simulink model "TorqueVectoring_6_1"  (R2023a)
settings: Solver=FixedStepAuto  StartTime=0.0  StopTime=8  FixedStep=.001  RelTol=1e-3
model workspace (MAT data in the model file):
  slipTarget = Simulink.Parameter
  slipTarget.Value = 20
  slipTarget.DataType = 'auto'
  slipTarget.Complexity = 'real'
  slipTarget.Dimensions = [1 1]
values from neighbouring files (symbols this model uses):
  Kd_slip = 0    [Main_TorqueVectoring_5_1.m]
  Kd_yaw = 0    [Main_TorqueVectoring_5_1.m]
  Ki_slip = 50    [Main_TorqueVectoring_5_1.m]
  Ki_yaw = 10    [Main_TorqueVectoring_5_1.m]
  Kp_slip = 250    [Main_TorqueVectoring_5_1.m]
  Kp_yaw = 100    [Main_TorqueVectoring_5_1.m]
  slip_windupLower = -inf    [Main_TorqueVectoring_5_1.m]
  slip_windupUpper = inf    [Main_TorqueVectoring_5_1.m]
  slipTarget = .2    (= 0.2)    [Main_TorqueVectoring_5_1.m]
  steering = table2array(yawrateSteering)    [Main_TorqueVectoring_5_1.m]
  yaw_prev_error = 0    [Main_TorqueVectoring_5_1.m]
  yawRate = table2array(yawrateTable)    [Main_TorqueVectoring_5_1.m]
  yawrateVelocity = [0, 5, 10, 15, 20, 25, 30, 35]    [Main_TorqueVectoring_5_1.m]
undefined symbols (not defined in the file or in its folder): sigbuilder_block, VehicleVelocity
libraries: slpidlib x6
(part 1 of 4)
settings Model: Creator=jwong  LastModifiedBy=melis
settings OptimizationCC: ReuseModelBlockBuffer=off
settings DebuggingCC: IgnoredZcDiagnostic=none
settings ModelReferenceCC: EnableRefExpFcnMdlSchedulingChecks=on

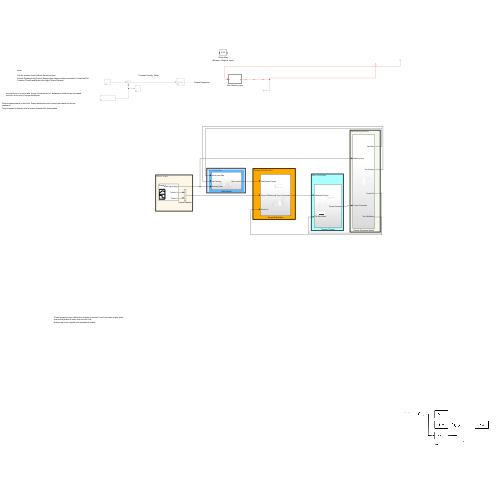
[thumbnail: Simulink's stored preview of the top-level diagram]
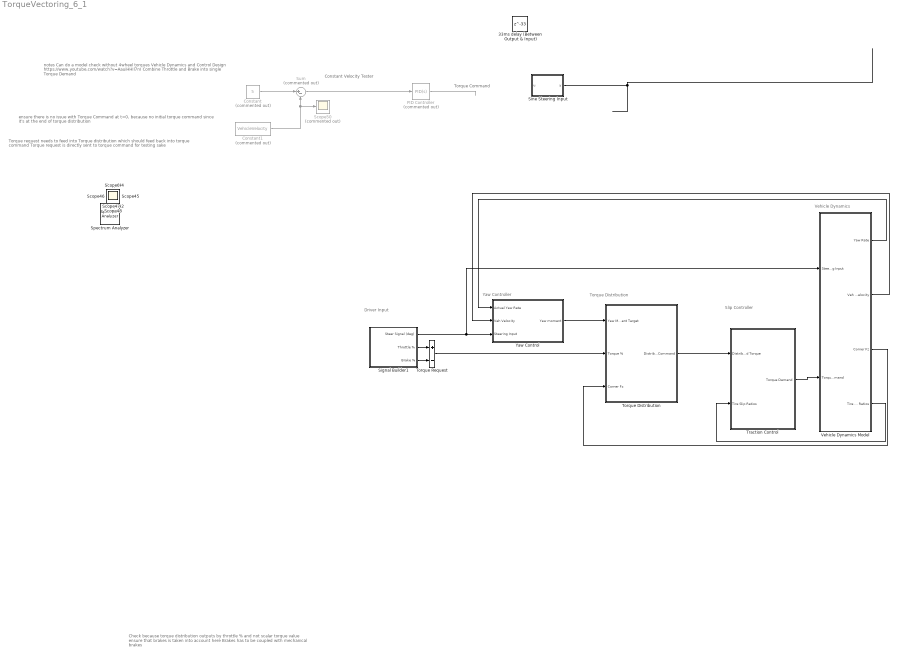
== system TorqueVectoring_6_1 ==
  note: Check because torque distribution outputs by throttle % and not scalar torque value
      | ensure that brakes is taken into account here
      | Brakes has to be coupled with mechanical brakes
  note: Driver Input
  note: Slip Controller
  note: ensure there is no issue with Torque Command at t=0, because no initial torque command since it's at the end of torque distribution
  note: Torque Command
  note: Constant Velocity Tester
  note: Torque request needs to feed into Torque distribution which should feed back into torque command
      | Torque request is directly sent to torque command for testing sake
  note: notes
      |
      | Can do a model check without 4wheel torques
      | Vehicle Dynamics and Control Design https://www.youtube.com/watch?v=AauiHHIl7nI
      | Combine Throttle and Brake into single Torque Demand
  note: Yaw Controller
  note: Torque Distribution
  note: Vehicle Dynamics
  33ms delay (Between Output & Input) : Delay  DelayLength=33
  Constant : Constant  Commented=on  Value=5
  Constant1 : Constant  Commented=on  Value=VehicleVelocity
  PID Controller : slpidlib/PID Controller  Commented=on  Controller=PID  Form=Parallel  TimeDomain=Continuous-time  UseExternalTs=off  SampleTime=-1  IntegratorMethod=Forward Euler  FilterMethod=Forward Euler  ControllerParametersSource=internal  P=1  I=1  UseKiTs=off  D=0  N=100  UseFilter=on  TunerSelectOption=Transfer Function Based (PID Tuner App)  InitialConditionSource=internal  InitialConditionForIntegrator=0  InitialConditionForFilter=0  DifferentiatorICPrevScaledInput=0  ExternalReset=none  TrackingMode=off  Kt=1  LimitOutput=off  SatLimitsSource=internal  UpperSaturationLimit=inf  LowerSaturationLimit=-inf  LinearizeAsGain=on  AntiWindupMode=none  Kb=1  LimitIntegrator=off  UpperIntegratorSaturationLimit=inf  LowerIntegratorSaturationLimit=-inf  POutMin=[]  POutMax=[]  IOutMin=[]  IOutMax=[]  DOutMin=[]  DOutMax=[]  NOutMin=[]  NOutMax=[]  SumOutMin=[]  SumOutMax=[]  SaturationOutMin=[]  SaturationOutMax=[]  PParamMin=[]  PParamMax=[]  IParamMin=[]  IParamMax=[]  DParamMin=[]  DParamMax=[]  NParamMin=[]  NParamMax=[]  KbParamMin=[]  KbParamMax=[]  KtParamMin=[]  KtParamMax=[]  KbOutMin=[]  KbOutMax=[]  KtOutMin=[]  KtOutMax=[]  IntegratorOutMin=[]  IntegratorOutMax=[]  FilterOutMin=[]  FilterOutMax=[]  SumI1OutMin=[]  SumI1OutMax=[]  SumI2OutMin=[]  SumI2OutMax=[]  SumI3OutMin=[]  SumI3OutMax=[]  SumI4OutMin=[]  SumI4OutMax=[]  SumDOutMin=[]  SumDOutMax=[]  DifferentiatorOutMin=[]  DifferentiatorOutMax=[]  FilterDiffOutCoefMin=[]  FilterDiffOutCoefMax=[]  ReciprocalOutMin=[]  ReciprocalOutMax=[]  SumDenOutMin=[]  SumDenOutMax=[]  SumNumOutMin=[]  SumNumOutMax=[]  DivideOutMin=[]  DivideOutMax=[]  UdiffTsProdOutMin=[]  UdiffTsProdOutMax=[]  NTsProdOutMin=[]  NTsProdOutMax=[]  UintegralTsProdOutMin=[]  UintegralTsProdOutMax=[]  UngainTsProdOutMin=[]  UngainTsProdOutMax=[]  ClampingZeroOutDataTypeStr=Inherit: Inherit via back propagation  ClampingZeroOutMin=[]  ClampingZeroOutMax=[]  FilterDenConstantOutDataTypeStr=Inherit: Inherit via back propagation  FilterDenConstantOutMin=[]  FilterDenConstantOutMax=[]  PCopyOutDataTypeStr=Inherit: Inherit via back propagation  PCopyOutMin=[]  PCopyOutMax=[]  NCopyOutDataTypeStr=Inherit: Inherit via back propagation  NCopyOutMin=[]  NCopyOutMax=[]  IntegratorContinuousStateAttributes=''  IntegratorStateMustResolveToSignalObject=off  IntegratorRTWStateStorageClass=Auto  FilterContinuousStateAttributes=''  FilterStateMustResolveToSignalObject=off  FilterRTWStateStorageClass=Auto  ParallelPVariant=InternalParameters  IdealPVariant=Disabled  IVariant=InternalParameters  DVariant=InternalParameters  IntegratorVariant=Continuous  SatVariant=Disabled  AWVariant=Passthrough  PCopyVariant=Disabled  TRVariant=Disabled  FdbkBlocksVariant=Forward  IdealPFdbkVariant=Disabled  SatFdbkVariant=Disabled  DerivativeFilterVariant=ContFilter  NVariant=InternalParameters  NCopyVariant=Disabled  FilterICVariant=InternalICsFilter  IntegratorICVariant=InternalICs  ExternalResetVariant=Disabled  TRSumVariant=Passthrough  SumFdbkVariant=Disabled  SumVariant=Sum_PID  TsampFilterVariant=InternalTs  TsampNgainVariant=Passthrough  TsampIntegralVariant=Disabled_SignalSpec  ExternalSaturationOutDataTypeStr=Inherit: Same as second input
  Scope50 : Scope  Commented=on
  Signal Builder1 : Subsystem  Tag=STV Subsys  LoadFcn=sigbuilder_block('load');  StartFcn=sigbuilder_block('start');  StopFcn=sigbuilder_block('stop');  ClipboardFcn=sigbuilder_block('clipboard');  mask(Sigbuilder block){tuvar=[0:10]}
      mask help: Sigbuilder GUI
      mask init:
      | if ~strcmp(get_param(bdroot(gcbh),'SimulationStatus'),'stopped') tuvar = sigbuilder_block('maskInit'); end
      settings: CopyFcn=sigbuilder_block('copy');  DeleteFcn=sigbuilder_block('delete');  ModelCloseFcn=sigbuilder_block('modelClose');  PreSaveFcn=sigbuilder_block('preSave');  PauseFcn=sigbuilder_block('pause')  ContinueFcn=sigbuilder_block('continue')  NameChangeFcn=sigbuilder_block('namechange');  OpenFcn=sigbuilder_block('open',[120.75 66 1313.25 670.5 ]);  CloseFcn=sigbuilder_block('close');
      mask Display: plot(0, 0, 100, 100,[2, 2, 32, 32, 2], [68, 8, 8, 68, 68],[32, 2], [38, 38], [32, 19, 2],[53, 60, 44], [32, 17, 17, 2],[16, 16, 31, 31]);txt = getActiveGroup(gcbh);text(2, 100, txt,'verticalAlignment', 'top');
  Sine Steering Input : MATLAB Function  TreatAsAtomicUnit=on
  Sum : Sum  Commented=on  Inputs=|+-
  Torque Distribution : Subsystem
  Torque Request : Sum  Inputs=+-
  Traction Control : Subsystem
  Vehicle Dynamics Model : Subsystem
  Yaw Control : Subsystem
  Scope{6,39..48} (11 alike) : Scope
  Spectrum Analyzer : SpectrumAnalyzer  IOType=viewer  WindowPosition=[680 330 560 420]  Method=Welch  SampleRate=10  AveragingMethod=Running
      settings: OpenAtSimulationStart=off
  wires:
  Signal Builder1/1(Steer Signal (deg)) -> Yaw Control/3(Steering Input), Vehicle Dynamics Model/1(Steering Input)
  Signal Builder1/3(Brake %) -> Torque Request/2
  Vehicle Dynamics Model/4(Tire Slip Ratios) -> Traction Control/2(Tire Slip Ratios)
  Vehicle Dynamics Model/1(Yaw Rate) -> Yaw Control/1(Actual Yaw Rate)
  Yaw Control/1(Yaw moment) -> Torque Distribution/1(Yaw Moment Target)
  Traction Control/1(Torque Demand) -> Vehicle Dynamics Model/2(Torque Command)
  Signal Builder1/2(Throttle %) -> Torque Request/1
  Torque Request/1 -> Torque Distribution/2(Torque %)
  Sum/1 -> PID Controller/1
  Constant/1 -> Sum/1
  Vehicle Dynamics Model/2(Veh Velocity) -> Yaw Control/2(Veh Velocity)
  PID Controller/1 -> ?
  Vehicle Dynamics Model/3(Corner Fz) -> Torque Distribution/3(Corner Fz)
  Constant1/1 -> Scope50/1, Sum/2
  ? -> Sine Steering Input/1(u)
  Sine Steering Input/1(y) -> ?
  Torque Distribution/1(Distributed Torque Command) -> Traction Control/1("Distributed Torque ")

== system TorqueVectoring_6_1/Signal Builder1 ==
  Demux : Demux  Tag=STV Demux  Outputs=3
      settings: DisplayOption=none
  FromWs : FromWorkspace  Tag=STV FromWs  VariableName=tuvar
      SigBuilderData=|
      | common.afterFinalStr = 'Extrapolate'
      | common.sampleTime = 0
      | dataSet.timeRange = [0 30]
      | dataSet.name = 'Group 1'
      | sbobj.Name = 'Signal Builder'
      | sbobj.Groups.Name = 'Group 1'
      | sbobj.Groups.Signals(1).Name = 'Steer Signal (deg)'
      | sbobj.Groups.Signals(1).XData = [0 2 2 30]
      | sbobj.Groups.Signals(1).YData = [0 0 20 20]
      | sbobj.Groups.Signals(2).Name = 'Throttle %'
      | sbobj.Groups.Signals(2).XData = [0 2 30]
      | sbobj.Groups.Signals(2).YData = [85 85 85]
      | sbobj.Groups.Signals(3).Name = 'Brake %'
      | sbobj.Groups.Signals(3).XData = [0 5 30]
      | sbobj.Groups.Signals(3).YData = [0 0 0]
      | sbobj.Groups.TimeRange = [0 30]
  Steer Signal (deg) : Outport  Tag=STV Outport
  Throttle % : Outport  Tag=STV Outport  Port=2
  Brake % : Outport  Tag=STV Outport  Port=3
  wires:
  FromWs/1 -> Demux/1
  Demux/1 -> Steer Signal (deg)/1
  Demux/2 -> Throttle %/1
  Demux/3 -> Brake %/1

== system TorqueVectoring_6_1/Torque Distribution ==
  note: Throttle % needs to be checked against look up table and slip control for the maximum torque wheel
  note: output of saturation is the max torque requests for 4 tires, but driver Request is 1 signal
  note: FIX: The input is 4 signal mux of each corner max
  note: saturation can be used to set the limits to allowable torque
  note: Needs to switch based off a corner that has the maximum traction
  note: note
      | make sure this does not limit torque if slip control is not active
  note: note
      | Sum of Moments = (Tfl + Tfr + Trl + Trr)*tw/2/Rw
      | Max allowable torque - every other torque will be a percentage of that torque to = the yaw moment,
      |
      | if traction control = 1
      | torqueOutput = slipcontrolledTorque
      | elseif traction control = 0
      | torqueOutputMax = driverrequested torque% * maxTorqueallowable
      |
      | How to get max torque allowable to one wheel and distribute, by percentage?
      | Send peak torque to highest gripped outside tires, calculate torque that must be offset by other motors
  Yaw Moment Target : Inport
  Torque % : Inport  Port=2
  Corner Fz : Inport  Port=3
  Demux : Demux
  Front-Rear Bias : MATLAB Function  TreatAsAtomicUnit=on
  MATLAB Function : MATLAB Function  Commented=on  TreatAsAtomicUnit=on
  Mux : Mux
  Percentage : Gain  Gain=.01
  To Workspace1 : ToWorkspace  VariableName=distributedtorqueFL  SampleTime=-1
  To Workspace2 : ToWorkspace  VariableName=distributedtorqueFR  SampleTime=-1
  To Workspace3 : ToWorkspace  VariableName=distributedtorqueRL  SampleTime=-1
  To Workspace4 : ToWorkspace  VariableName=distributedtorqueRR  SampleTime=-1
  To Workspace9 : ToWorkspace  VariableName=TorquePer  SaveFormat=Timeseries  SampleTime=-1
  Torque Distribution : MATLAB Function  TreatAsAtomicUnit=on
  Distributed Torque Command : Outport
  wires:
  Yaw Moment Target/1 -> Torque Distribution/1(Mz)
  Corner Fz/1 -> Demux/1
  Demux/1 -> Front-Rear Bias/1(zFL)
  Demux/2 -> Front-Rear Bias/2(zFR)
  Demux/3 -> Front-Rear Bias/3(zRL)
  Demux/4 -> Front-Rear Bias/4(zRR)
  Front-Rear Bias/1(lambda) -> Torque Distribution/3(lambda)
  Torque %/1 -> Percentage/1
  Torque Distribution/2(FRtorque) -> To Workspace2/1, Mux/2
  Torque Distribution/3(RLtorque) -> To Workspace3/1, Mux/3
  Percentage/1 -> To Workspace9/1, Torque Distribution/2(torquePer)
  Mux/1 -> Distributed Torque Command/1
  Torque Distribution/1(FLtorque) -> To Workspace1/1, Mux/1
  Torque Distribution/4(RRtorque) -> To Workspace4/1, Mux/4

== system TorqueVectoring_6_1/Traction Control ==
  note: Outputs are converted to torque instead of tractive force because VCU will command torque setpoints to the inverters
  note: note
      | can bias front to have less torque output @ acceleration to ensure slip ratio and vice versa
  note: Torques must be split here because each tire has their own feedback
  note: note
      | if |slip ratio| > slip ratio target
      | Max allowable torque would be fed from lookup tables
  note: note
      | Does 4 PID Controllers make sense here?
      | Yes - slip control at each individual wheel depending on their indivudal slip
      | Does the PID output a torque command here?
      | Need slip ratio to work under braking - slip ratio target needs to be upper and lower bound
      | if torque command is negative, slip ratio target =-2
      | slip ratio is negative, cannot be > -2
  note: Slip target is a parameter variable of Model workspace
      | *see Model Explorer
  note: **Look up tables can be an an issue when slip ratio is 0 and therefore produces no load
  note: **Ensure Lookup tables can handle negative direction
  "Distributed Torque " : Inport
  Tire Slip Ratios : Inport  Port=2
  Add : Sum
  Demux : Demux
  FL : Subsystem
  FR : Subsystem
  Gain1 : Gain  Gain=1/1.2
  Mux : Mux
  RL : Subsystem
  RR : Subsystem
  Slip Target Constant : Constant  Value=slipTarget
  To Workspace4 : ToWorkspace  VariableName=torqueDemand  SampleTime=-1
  Torque Demand : Outport
  wires:
  Demux/1 -> FL/1(slip Ratio)
  Demux/2 -> FR/1(slip Ratio)
  Demux/3 -> RL/1(slip Ratio)
  Demux/4 -> RR/1(slip Ratio)
  Mux/1 -> Add/2, To Workspace4/1
  FL/1(Allowable Torque) -> Mux/1  "FL PID torque adjust"
  FR/1(Allowable Torque) -> Mux/2  "FR PID torque  adjust"
  RL/1(Allowable Torque) -> Mux/3  "RL PID torque adjust"
  RR/1(Allowable Torque) -> Mux/4  "RR PID torque  adjust"
  Slip Target Constant/1 -> RR/2(slipTarget), RL/2(slipTarget), FR/2(slipTarget), FL/2(slipTarget)
  Add/1 -> Torque Demand/1
  "Distributed Torque "/1 -> Add/1
  Tire Slip Ratios/1 -> Gain1/1
  Gain1/1 -> Demux/1

== system TorqueVectoring_6_1/Vehicle Dynamics Model ==
  note: Tire slipAngles not used to calculate Fy, not accurate enough sensors for real use
  Steering Input : Inport
  Torque Command : Inport  Port=2
  " Slip Angles" : Mux  Commented=on
  " Slip Ratios" : Mux
  14 DOF MODEL : Subsystem  mask{Ms=180.9, a=0.8169783, b=0.707009, wf=1.34, wr=1.34, h=0.23, mt=241.7, Lf=.64, Lr=.88392, Ip=64.46, Ir=15.34, Jz=70.38, mufl=7.4, mufr=7.4, murl=7.8, murr=7.8, Rw=.4064, Iw=3.033213, Ksfl=19.3, Ksfr=19.3, Ksrl=24.8, Ksrr=24.8, Csfl=1437.611, Csfr=1437.611, Csrl=1644.42, Csrr=1644.42, Ktfl=113832.44275, Ktfr=113832.44275, Ktrl=113832.44275, Ktrr=113832.44275, g=9.8}
      mask prompts: Ms "Vehicle sprung mass (kg)"; a "Distance of sprung mass C.G. from front axle (m)"; b "Distance of sprung mass C.G. from rear axle (m)"; wf "Front track width (m)"; wr "Rear track width (m)"; h "Height of sprung mass C.G. from rground (m)"; mt "Vehicle total mass (kg)"; Lf "Distance of vehicle C.G. from front axle (m)"; Lr "Distance of vehicle C.G. from rear axle (m)"; Ip "Pitch moment of inertia (kgm^2)"; Ir "Roll moment of inertia (kgm^2)"; Jz "Yaw moment of inertia (kgm^2)"; mufl "Front left unsprung mass (kg)"; mufr "Front right unsprung mass (kg)"; murl "Rear left unsprung mass (kg)"; murr "Rear right unsprung mass (kg)"; Rw "Wheel radius (m)"; Iw "Wheel moment of inertia (kgm^2)"; Ksfl "Front left suspension stiffness (N/m)"; Ksfr "Front right suspension stiffness (N/m)"; Ksrl "Rear left suspension stiffness (N/m)"; Ksrr "Rear right suspension stiffness (N/m)"; Csfl "Front left suspension damping coefficient (Nsec/m)"; Csfr "Front right suspension damping coefficient (Nsec/m)"; Csrl "Rear left suspension damping coefficient (Nsec/m)"; Csrr "Rear right suspension damping coefficient (Nsec/m)"; Ktfl "Front left tire stiffness (N/m)"; Ktfr "Front right tire stiffness (N/m)"; Ktrl "Rear left tire stiffness (N/m)"; Ktrr "Rear right tire stiffness (N/m)"; g "Gravitational acceleration (ms^-2)"
      mask Display: %image(imread('E:\Google Drive\FSAE Electric\In Hub Motors Torque Vectoring Masters Project\Simulink\IMG_8647.JPG'))
  Constant : Constant  Value=.001
  Demux : Demux
  Gain : Gain
  Gain1 : Gain  Gain=1/1000
  Radians to deg : Gain  Gain=57.2958
  Scope : Scope
  Signal Builder : Subsystem  Tag=STV Subsys  LoadFcn=sigbuilder_block('load');  StartFcn=sigbuilder_block('start');  StopFcn=sigbuilder_block('stop');  ClipboardFcn=sigbuilder_block('clipboard');  mask(Sigbuilder block){tuvar=[0:10]}
      mask help: Simulink:masks:SigbuilderBlock_MD
      mask init:
      | if ~strcmp(get_param(bdroot(gcbh),'SimulationStatus'),'stopped') tuvar = sigbuilder_block('maskInit'); end
      settings: CopyFcn=sigbuilder_block('copy');  DeleteFcn=sigbuilder_block('delete');  ModelCloseFcn=sigbuilder_block('modelClose');  PreSaveFcn=sigbuilder_block('preSave');  PauseFcn=sigbuilder_block('pause');  ContinueFcn=sigbuilder_block('continue');  NameChangeFcn=sigbuilder_block('namechange');  OpenFcn=sigbuilder_block('open',[437.6 199.2 550.4 400 ]);  CloseFcn=sigbuilder_block('close');
      mask Display: plot(0, 0, 100, 100,[2, 2, 32, 32, 2], [68, 8, 8, 68, 68],[32, 2], [38, 38], [32, 19, 2],[53, 60, 44], [32, 17, 17, 2],[16, 16, 31, 31]);txt = getActiveGroup(gcbh);text(2, 100, txt,'verticalAlignment', 'top');
  To Workspace : ToWorkspace  VariableName=LatAcc  SampleTime=-1
  To Workspace1 : ToWorkspace  VariableName=YawRate  SampleTime=-1
  To Workspace5 : ToWorkspace  VariableName=T_FL  SampleTime=-1
  To Workspace6 : ToWorkspace  VariableName=T_FR  SampleTime=-1
  To Workspace7 : ToWorkspace  VariableName=T_RL  SampleTime=-1
  To Workspace8 : ToWorkspace  VariableName=T_RR  SampleTime=-1
  X Position : ToWorkspace  VariableName=X  SampleTime=-1
  Y Position : ToWorkspace  VariableName=Y  SampleTime=-1
  fl Slip : ToWorkspace  VariableName=FLsr  SampleTime=-1
  fl slip angle : Scope
  fr Slip : ToWorkspace  VariableName=FRsr  SampleTime=-1
  fr slip angle : Scope
  lateral acceleration : Scope
  rl Slip : ToWorkspace  VariableName=RLsr  SampleTime=-1
  rl slip angle : Scope
  roll angle : Scope
  rr Slip : ToWorkspace  VariableName=RRsr  SampleTime=-1
  rr slip angle : Scope
  steering : Scope
  yaw rate : Scope
  Yaw Rate : Outport
  Veh Velocity : Outport  Port=2
  Corner Fz : Outport  Port=3
  Tire Slip Ratios : Outport  Port=4
  wires:
  14 DOF MODEL/3(roll angle) -> roll angle/1
  14 DOF MODEL/1(ay) -> To Workspace/1, lateral acceleration/1
  Gain/1 -> 14 DOF MODEL/1(steer)
  14 DOF MODEL/9(Y) -> Y Position/1  "Ypos"
  14 DOF MODEL/8(X) -> X Position/1  "Xpos"
  Steering Input/1 -> steering/1, Gain/1
  14 DOF MODEL/2(yaw rate) -> Radians to deg/1
  14 DOF MODEL/4(fl slip angle) -> " Slip Angles"/1, fl slip angle/1
  14 DOF MODEL/5(fr slip angle) -> " Slip Angles"/2, fr slip angle/1
  14 DOF MODEL/6(rl slip angle) -> " Slip Angles"/3, rl slip angle/1
  14 DOF MODEL/7(rr slip angle) -> " Slip Angles"/4, rr slip angle/1
  14 DOF MODEL/11(fr Slip Ratio) -> fr Slip/1, " Slip Ratios"/2  "fr SlipRatio"
  14 DOF MODEL/12(rl Slip Ratio) -> " Slip Ratios"/3, rl Slip/1  "rl SlipRatio"
  " Slip Ratios"/1 -> Gain1/1
  14 DOF MODEL/10(fl Slip Ratio) -> fl Slip/1, " Slip Ratios"/1  "fl SlipRatio"
  14 DOF MODEL/13(rr Slip Ratio) -> rr Slip/1, " Slip Ratios"/4  "rr SlipRatio"
  " Slip Angles"/1 -> ?
  Torque Command/1 -> Demux/1, Scope/1
  Constant/1 -> 14 DOF MODEL/2(Vx (Initial))
  Radians to deg/1 -> Yaw Rate/1, yaw rate/1, To Workspace1/1  "deg"
  14 DOF MODEL/14(Veh Velocity) -> Veh Velocity/1
  14 DOF MODEL/15(Corner Fz) -> Corner Fz/1
  Demux/3 -> To Workspace7/1, 14 DOF MODEL/5(TaRL)
  Demux/2 -> To Workspace6/1, 14 DOF MODEL/4(TaFR)
  Demux/4 -> To Workspace8/1, 14 DOF MODEL/6(TaRR)
  Demux/1 -> To Workspace5/1, 14 DOF MODEL/3(TaFL)
  Gain1/1 -> Tire Slip Ratios/1

== system TorqueVectoring_6_1/Yaw Control ==
  Actual Yaw Rate : Inport
  Veh Velocity : Inport  Port=2
  Steering Input : Inport  Port=3
  Abs : Abs  SaturateOnIntegerOverflow=off
  Add : Sum
  Constant : Constant  Value=.001
  Constant1 : Constant  Value=10
  Constant2 : Constant  Value=-1
  Gain : Gain  Gain=1.6180217600198381947242800905118
  MATLAB Function : MATLAB Function  TreatAsAtomicUnit=on
  PID Controller : slpidlib/PID Controller  Commented=on  Controller=PID  Form=Parallel  TimeDomain=Discrete-time  UseExternalTs=off  SampleTime=-1  IntegratorMethod=Backward Euler  FilterMethod=Backward Euler  ControllerParametersSource=internal  P=Kp_yaw  I=Ki_yaw  UseKiTs=off  D=Kd_yaw  N=100  UseFilter=on  TunerSelectOption=Frequency Response Based  InitialConditionSource=internal  InitialConditionForIntegrator=0  InitialConditionForFilter=0  DifferentiatorICPrevScaledInput=0  ExternalReset=none  TrackingMode=off  Kt=1  LimitOutput=on  SatLimitsSource=internal  UpperSaturationLimit=inf  LowerSaturationLimit=-inf  LinearizeAsGain=on  AntiWindupMode=clamping  Kb=1  LimitIntegrator=off  UpperIntegratorSaturationLimit=inf  LowerIntegratorSaturationLimit=-inf  POutMin=[]  POutMax=[]  IOutMin=[]  IOutMax=[]  DOutMin=[]  DOutMax=[]  NOutMin=[]  NOutMax=[]  SumOutMin=[]  SumOutMax=[]  SaturationOutMin=[]  SaturationOutMax=[]  PParamMin=[]  PParamMax=[]  IParamMin=[]  IParamMax=[]  DParamMin=[]  DParamMax=[]  NParamMin=[]  NParamMax=[]  KbParamMin=[]  KbParamMax=[]  KtParamMin=[]  KtParamMax=[]  KbOutMin=[]  KbOutMax=[]  KtOutMin=[]  KtOutMax=[]  IntegratorOutMin=[]  IntegratorOutMax=[]  FilterOutMin=[]  FilterOutMax=[]  SumI1OutMin=[]  SumI1OutMax=[]  SumI2OutMin=[]  SumI2OutMax=[]  SumI3OutMin=[]  SumI3OutMax=[]  SumI4OutMin=[]  SumI4OutMax=[]  SumDOutMin=[]  SumDOutMax=[]  DifferentiatorOutMin=[]  DifferentiatorOutMax=[]  FilterDiffOutCoefMin=[]  FilterDiffOutCoefMax=[]  ReciprocalOutMin=[]  ReciprocalOutMax=[]  SumDenOutMin=[]  SumDenOutMax=[]  SumNumOutMin=[]  SumNumOutMax=[]  DivideOutMin=[]  DivideOutMax=[]  UdiffTsProdOutMin=[]  UdiffTsProdOutMax=[]  NTsProdOutMin=[]  NTsProdOutMax=[]  UintegralTsProdOutMin=[]  UintegralTsProdOutMax=[]  UngainTsProdOutMin=[]  UngainTsProdOutMax=[]  ClampingZeroOutDataTypeStr=Inherit: Inherit via back propagation  ClampingZeroOutMin=[]  ClampingZeroOutMax=[]  FilterDenConstantOutDataTypeStr=Inherit: Inherit via back propagation  FilterDenConstantOutMin=[]  FilterDenConstantOutMax=[]  PCopyOutDataTypeStr=Inherit: Inherit via back propagation  PCopyOutMin=[]  PCopyOutMax=[]  NCopyOutDataTypeStr=Inherit: Inherit via back propagation  NCopyOutMin=[]  NCopyOutMax=[]  IntegratorContinuousStateAttributes=''  IntegratorStateMustResolveToSignalObject=off  IntegratorRTWStateStorageClass=Auto  FilterContinuousStateAttributes=''  FilterStateMustResolveToSignalObject=off  FilterRTWStateStorageClass=Auto  ParallelPVariant=InternalParameters  IdealPVariant=Disabled  IVariant=InternalParameters  DVariant=InternalParameters  IntegratorVariant=Discrete  SatVariant=Enabled  AWVariant=DiscClampingParallel  PCopyVariant=Disabled  TRVariant=Disabled  FdbkBlocksVariant=Feedback  IdealPFdbkVariant=Passthrough  SatFdbkVariant=Passthrough  DerivativeFilterVariant=BackwardEulerFilter  NVariant=InternalParameters  NCopyVariant=InternalParameters  FilterICVariant=InternalICsFilter  IntegratorICVariant=InternalICs  ExternalResetVariant=Disabled  TRSumVariant=Passthrough  SumFdbkVariant=Enabled  SumVariant=Sum_PID  TsampFilterVariant=InternalTs  TsampNgainVariant=Passthrough  TsampIntegralVariant=Disabled_SignalSpec  ExternalSaturationOutDataTypeStr=Inherit: Same as second input
  Product2 : Product
  Steering vs Velocity Yaw Rate Lookup Table : Lookup_n-D  BreakpointsForDimension1=steering  BreakpointsForDimension2=yawrateVelocity  Table=yawRate  InternalRulePriority=Speed  RndMeth=Simplest
      settings: InputPortMap=u0,u1
  Sum : Sum  Inputs=|+-
  Switch : Switch  Criteria=u2 > Threshold  ZeroCross=off  SaturateOnIntegerOverflow=off  InputSameDT=off
  To Workspace : ToWorkspace  VariableName=steeringAngle  SaveFormat=Timeseries  SampleTime=-1
  To Workspace1 : ToWorkspace  VariableName=YawRateSetpoint  SaveFormat=Timeseries  SampleTime=-1
  To Workspace2 : ToWorkspace  VariableName=YawMomentTarget  SaveFormat=Timeseries  SampleTime=-1
  To Workspace3 : ToWorkspace  VariableName=YawRateError  SaveFormat=Timeseries  SampleTime=-1
  Yaw moment : Outport
  wires:
  Steering Input/1 -> To Workspace/1, Switch/2, Product2/1, Abs/1
  Sum/1 -> To Workspace3/1, MATLAB Function/1(yaw_error)  "Yaw Rate Error"
  Veh Velocity/1 -> Add/1
  Steering vs Velocity Yaw Rate Lookup Table/1 -> Gain/1  "Yaw Rate  Setpoint"
  Add/1 -> Steering vs Velocity Yaw Rate Lookup Table/2
  Constant/1 -> Add/2
  Abs/1 -> Steering vs Velocity Yaw Rate Lookup Table/1
  Constant2/1 -> Product2/2
  Product2/1 -> Switch/3
  Switch/1 -> Yaw moment/1
  Actual Yaw Rate/1 -> Sum/2
  Gain/1 -> To Workspace1/1, Sum/1
  MATLAB Function/1(yaw_target) -> To Workspace2/1, Switch/1

== system TorqueVectoring_6_1/Traction Control/FL ==
  slip Ratio : Inport
  slipTarget : Inport  Port=2
  Constant : Constant  Value=0
  MATLAB Function : MATLAB Function  TreatAsAtomicUnit=on
  PID Controller5 : slpidlib/PID Controller  Controller=PID  Form=Parallel  TimeDomain=Continuous-time  UseExternalTs=off  SampleTime=-1  IntegratorMethod=Forward Euler  FilterMethod=Forward Euler  ControllerParametersSource=internal  P=Kp_slip  I=Ki_slip  UseKiTs=off  D=Kd_slip  N=100  UseFilter=on  TunerSelectOption=Transfer Function Based (PID Tuner App)  ZeroCross=off  InitialConditionSource=internal  InitialConditionForIntegrator=0  InitialConditionForFilter=0  DifferentiatorICPrevScaledInput=0  ExternalReset=none  TrackingMode=off  Kt=1  LimitOutput=off  SatLimitsSource=internal  UpperSaturationLimit=slip_windupUpper  LowerSaturationLimit=slip_windupLower  LinearizeAsGain=on  AntiWindupMode=clamping  Kb=1  LimitIntegrator=off  UpperIntegratorSaturationLimit=inf  LowerIntegratorSaturationLimit=-inf  POutMin=[]  POutMax=[]  IOutMin=[]  IOutMax=[]  DOutMin=[]  DOutMax=[]  NOutMin=[]  NOutMax=[]  SumOutMin=[]  SumOutMax=[]  SaturationOutMin=[]  SaturationOutMax=[]  PParamMin=[]  PParamMax=[]  IParamMin=[]  IParamMax=[]  DParamMin=[]  DParamMax=[]  NParamMin=[]  NParamMax=[]  KbParamMin=[]  KbParamMax=[]  KtParamMin=[]  KtParamMax=[]  KbOutMin=[]  KbOutMax=[]  KtOutMin=[]  KtOutMax=[]  IntegratorOutMin=[]  IntegratorOutMax=[]  FilterOutMin=[]  FilterOutMax=[]  SumI1OutMin=[]  SumI1OutMax=[]  SumI2OutMin=[]  SumI2OutMax=[]  SumI3OutMin=[]  SumI3OutMax=[]  SumI4OutMin=[]  SumI4OutMax=[]  SumDOutMin=[]  SumDOutMax=[]  DifferentiatorOutMin=[]  DifferentiatorOutMax=[]  FilterDiffOutCoefMin=[]  FilterDiffOutCoefMax=[]  ReciprocalOutMin=[]  ReciprocalOutMax=[]  SumDenOutMin=[]  SumDenOutMax=[]  SumNumOutMin=[]  SumNumOutMax=[]  DivideOutMin=[]  DivideOutMax=[]  UdiffTsProdOutMin=[]  UdiffTsProdOutMax=[]  NTsProdOutMin=[]  NTsProdOutMax=[]  UintegralTsProdOutMin=[]  UintegralTsProdOutMax=[]  UngainTsProdOutMin=[]  UngainTsProdOutMax=[]  ClampingZeroOutDataTypeStr=Inherit: Inherit via back propagation  ClampingZeroOutMin=[]  ClampingZeroOutMax=[]  FilterDenConstantOutDataTypeStr=Inherit: Inherit via back propagation  FilterDenConstantOutMin=[]  FilterDenConstantOutMax=[]  PCopyOutDataTypeStr=Inherit: Inherit via back propagation  PCopyOutMin=[]  PCopyOutMax=[]  NCopyOutDataTypeStr=Inherit: Inherit via back propagation  NCopyOutMin=[]  NCopyOutMax=[]  IntegratorContinuousStateAttributes=''  IntegratorStateMustResolveToSignalObject=off  IntegratorRTWStateStorageClass=Auto  FilterContinuousStateAttributes=''  FilterStateMustResolveToSignalObject=off  FilterRTWStateStorageClass=Auto  ParallelPVariant=InternalParameters  IdealPVariant=Disabled  IVariant=InternalParameters  DVariant=InternalParameters  IntegratorVariant=Continuous  SatVariant=Disabled  AWVariant=Passthrough  PCopyVariant=Disabled  TRVariant=Disabled  FdbkBlocksVariant=Forward  IdealPFdbkVariant=Disabled  SatFdbkVariant=Disabled  DerivativeFilterVariant=ContFilter  NVariant=InternalParameters  NCopyVariant=Disabled  FilterICVariant=InternalICsFilter  IntegratorICVariant=InternalICs  ExternalResetVariant=Disabled  TRSumVariant=Passthrough  SumFdbkVariant=Disabled  SumVariant=Sum_PID  TsampFilterVariant=InternalTs  TsampNgainVariant=Passthrough  TsampIntegralVariant=Disabled_SignalSpec  ExternalSaturationOutDataTypeStr=Inherit: Same as second input
  Scope : Scope
  Scope1 : Scope
  Sum5 : Sum  Inputs=|+-
  Switch : Switch  Criteria=u2 > Threshold  ZeroCross=off  SaturateOnIntegerOverflow=off  InputSameDT=off
  To Workspace1 : ToWorkspace  VariableName=FLslipError  SaveFormat=Timeseries  SampleTime=-1
  fl Slip : ToWorkspace  VariableName=FLsr1  SampleTime=-1
  Allowable Torque : Outport
  wires:
  MATLAB Function/2(setpoint) -> Sum5/1
  Sum5/1 -> To Workspace1/1, PID Controller5/1  "slip error"
  Switch/1 -> Allowable Torque/1
  slip Ratio/1 -> fl Slip/1, MATLAB Function/1(actualSlip), Sum5/2
  slipTarget/1 -> MATLAB Function/2(SlipTarget)
  MATLAB Function/1(enable) -> Switch/2, Scope/1
  PID Controller5/1 -> Scope1/1, Switch/1
  Constant/1 -> Switch/3

== system TorqueVectoring_6_1/Traction Control/FR ==
  slip Ratio : Inport
  slipTarget : Inport  Port=2
  Constant : Constant  Value=0
  MATLAB Function : MATLAB Function  TreatAsAtomicUnit=on
  PID Controller5 : slpidlib/PID Controller  Controller=PID  Form=Parallel  TimeDomain=Continuous-time  UseExternalTs=off  SampleTime=-1  IntegratorMethod=Forward Euler  FilterMethod=Forward Euler  ControllerParametersSource=internal  P=Kp_slip  I=Ki_slip  UseKiTs=off  D=Kd_slip  N=100  UseFilter=on  TunerSelectOption=Transfer Function Based (PID Tuner App)  ZeroCross=off  InitialConditionSource=internal  InitialConditionForIntegrator=0  InitialConditionForFilter=0  DifferentiatorICPrevScaledInput=0  ExternalReset=none  TrackingMode=off  Kt=1  LimitOutput=off  SatLimitsSource=internal  UpperSaturationLimit=slip_windupUpper  LowerSaturationLimit=slip_windupLower  LinearizeAsGain=on  AntiWindupMode=clamping  Kb=1  LimitIntegrator=off  UpperIntegratorSaturationLimit=inf  LowerIntegratorSaturationLimit=-inf  POutMin=[]  POutMax=[]  IOutMin=[]  IOutMax=[]  DOutMin=[]  DOutMax=[]  NOutMin=[]  NOutMax=[]  SumOutMin=[]  SumOutMax=[]  SaturationOutMin=[]  SaturationOutMax=[]  PParamMin=[]  PParamMax=[]  IParamMin=[]  IParamMax=[]  DParamMin=[]  DParamMax=[]  NParamMin=[]  NParamMax=[]  KbParamMin=[]  KbParamMax=[]  KtParamMin=[]  KtParamMax=[]  KbOutMin=[]  KbOutMax=[]  KtOutMin=[]  KtOutMax=[]  IntegratorOutMin=[]  IntegratorOutMax=[]  FilterOutMin=[]  FilterOutMax=[]  SumI1OutMin=[]  SumI1OutMax=[]  SumI2OutMin=[]  SumI2OutMax=[]  SumI3OutMin=[]  SumI3OutMax=[]  SumI4OutMin=[]  SumI4OutMax=[]  SumDOutMin=[]  SumDOutMax=[]  DifferentiatorOutMin=[]  DifferentiatorOutMax=[]  FilterDiffOutCoefMin=[]  FilterDiffOutCoefMax=[]  ReciprocalOutMin=[]  ReciprocalOutMax=[]  SumDenOutMin=[]  SumDenOutMax=[]  SumNumOutMin=[]  SumNumOutMax=[]  DivideOutMin=[]  DivideOutMax=[]  UdiffTsProdOutMin=[]  UdiffTsProdOutMax=[]  NTsProdOutMin=[]  NTsProdOutMax=[]  UintegralTsProdOutMin=[]  UintegralTsProdOutMax=[]  UngainTsProdOutMin=[]  UngainTsProdOutMax=[]  ClampingZeroOutDataTypeStr=Inherit: Inherit via back propagation  ClampingZeroOutMin=[]  ClampingZeroOutMax=[]  FilterDenConstantOutDataTypeStr=Inherit: Inherit via back propagation  FilterDenConstantOutMin=[]  FilterDenConstantOutMax=[]  PCopyOutDataTypeStr=Inherit: Inherit via back propagation  PCopyOutMin=[]  PCopyOutMax=[]  NCopyOutDataTypeStr=Inherit: Inherit via back propagation  NCopyOutMin=[]  NCopyOutMax=[]  IntegratorContinuousStateAttributes=''  IntegratorStateMustResolveToSignalObject=off  IntegratorRTWStateStorageClass=Auto  FilterContinuousStateAttributes=''  FilterStateMustResolveToSignalObject=off  FilterRTWStateStorageClass=Auto  ParallelPVariant=InternalParameters  IdealPVariant=Disabled  IVariant=InternalParameters  DVariant=InternalParameters  IntegratorVariant=Continuous  SatVariant=Disabled  AWVariant=Passthrough  PCopyVariant=Disabled  TRVariant=Disabled  FdbkBlocksVariant=Forward  IdealPFdbkVariant=Disabled  SatFdbkVariant=Disabled  DerivativeFilterVariant=ContFilter  NVariant=InternalParameters  NCopyVariant=Disabled  FilterICVariant=InternalICsFilter  IntegratorICVariant=InternalICs  ExternalResetVariant=Disabled  TRSumVariant=Passthrough  SumFdbkVariant=Disabled  SumVariant=Sum_PID  TsampFilterVariant=InternalTs  TsampNgainVariant=Passthrough  TsampIntegralVariant=Disabled_SignalSpec  ExternalSaturationOutDataTypeStr=Inherit: Same as second input
  Scope : Scope
  Scope1 : Scope
  Sum5 : Sum  Inputs=|+-
  Switch : Switch  Criteria=u2 > Threshold  ZeroCross=off  SaturateOnIntegerOverflow=off  InputSameDT=off
  To Workspace1 : ToWorkspace  VariableName=FRslipError  SaveFormat=Timeseries  SampleTime=-1
  fl Slip : ToWorkspace  VariableName=FRsr1  SampleTime=-1
  Allowable Torque : Outport
  wires:
  Constant/1 -> Switch/3
  slipTarget/1 -> MATLAB Function/2(SlipTarget)
  MATLAB Function/1(enable) -> Switch/2, Scope/1
  slip Ratio/1 -> fl Slip/1, MATLAB Function/1(actualSlip), Sum5/2
  Switch/1 -> Allowable Torque/1
  MATLAB Function/2(setpoint) -> Sum5/1
  Sum5/1 -> To Workspace1/1, PID Controller5/1  "slip error"
  PID Controller5/1 -> Scope1/1, Switch/1

== system TorqueVectoring_6_1/Traction Control/RL ==
  slip Ratio : Inport
  slipTarget : Inport  Port=2
  Constant : Constant  Value=0
  MATLAB Function : MATLAB Function  TreatAsAtomicUnit=on
  PID Controller5 : slpidlib/PID Controller  Controller=PID  Form=Parallel  TimeDomain=Continuous-time  UseExternalTs=off  SampleTime=-1  IntegratorMethod=Forward Euler  FilterMethod=Forward Euler  ControllerParametersSource=internal  P=Kp_slip  I=Ki_slip  UseKiTs=off  D=Kd_slip  N=100  UseFilter=on  TunerSelectOption=Transfer Function Based (PID Tuner App)  ZeroCross=off  InitialConditionSource=internal  InitialConditionForIntegrator=0  InitialConditionForFilter=0  DifferentiatorICPrevScaledInput=0  ExternalReset=none  TrackingMode=off  Kt=1  LimitOutput=off  SatLimitsSource=internal  UpperSaturationLimit=slip_windupUpper  LowerSaturationLimit=slip_windupLower  LinearizeAsGain=on  AntiWindupMode=clamping  Kb=1  LimitIntegrator=off  UpperIntegratorSaturationLimit=inf  LowerIntegratorSaturationLimit=-inf  POutMin=[]  POutMax=[]  IOutMin=[]  IOutMax=[]  DOutMin=[]  DOutMax=[]  NOutMin=[]  NOutMax=[]  SumOutMin=[]  SumOutMax=[]  SaturationOutMin=[]  SaturationOutMax=[]  PParamMin=[]  PParamMax=[]  IParamMin=[]  IParamMax=[]  DParamMin=[]  DParamMax=[]  NParamMin=[]  NParamMax=[]  KbParamMin=[]  KbParamMax=[]  KtParamMin=[]  KtParamMax=[]  KbOutMin=[]  KbOutMax=[]  KtOutMin=[]  KtOutMax=[]  IntegratorOutMin=[]  IntegratorOutMax=[]  FilterOutMin=[]  FilterOutMax=[]  SumI1OutMin=[]  SumI1OutMax=[]  SumI2OutMin=[]  SumI2OutMax=[]  SumI3OutMin=[]  SumI3OutMax=[]  SumI4OutMin=[]  SumI4OutMax=[]  SumDOutMin=[]  SumDOutMax=[]  DifferentiatorOutMin=[]  DifferentiatorOutMax=[]  FilterDiffOutCoefMin=[]  FilterDiffOutCoefMax=[]  ReciprocalOutMin=[]  ReciprocalOutMax=[]  SumDenOutMin=[]  SumDenOutMax=[]  SumNumOutMin=[]  SumNumOutMax=[]  DivideOutMin=[]  DivideOutMax=[]  UdiffTsProdOutMin=[]  UdiffTsProdOutMax=[]  NTsProdOutMin=[]  NTsProdOutMax=[]  UintegralTsProdOutMin=[]  UintegralTsProdOutMax=[]  UngainTsProdOutMin=[]  UngainTsProdOutMax=[]  ClampingZeroOutDataTypeStr=Inherit: Inherit via back propagation  ClampingZeroOutMin=[]  ClampingZeroOutMax=[]  FilterDenConstantOutDataTypeStr=Inherit: Inherit via back propagation  FilterDenConstantOutMin=[]  FilterDenConstantOutMax=[]  PCopyOutDataTypeStr=Inherit: Inherit via back propagation  PCopyOutMin=[]  PCopyOutMax=[]  NCopyOutDataTypeStr=Inherit: Inherit via back propagation  NCopyOutMin=[]  NCopyOutMax=[]  IntegratorContinuousStateAttributes=''  IntegratorStateMustResolveToSignalObject=off  IntegratorRTWStateStorageClass=Auto  FilterContinuousStateAttributes=''  FilterStateMustResolveToSignalObject=off  FilterRTWStateStorageClass=Auto  ParallelPVariant=InternalParameters  IdealPVariant=Disabled  IVariant=InternalParameters  DVariant=InternalParameters  IntegratorVariant=Continuous  SatVariant=Disabled  AWVariant=Passthrough  PCopyVariant=Disabled  TRVariant=Disabled  FdbkBlocksVariant=Forward  IdealPFdbkVariant=Disabled  SatFdbkVariant=Disabled  DerivativeFilterVariant=ContFilter  NVariant=InternalParameters  NCopyVariant=Disabled  FilterICVariant=InternalICsFilter  IntegratorICVariant=InternalICs  ExternalResetVariant=Disabled  TRSumVariant=Passthrough  SumFdbkVariant=Disabled  SumVariant=Sum_PID  TsampFilterVariant=InternalTs  TsampNgainVariant=Passthrough  TsampIntegralVariant=Disabled_SignalSpec  ExternalSaturationOutDataTypeStr=Inherit: Same as second input
  Scope : Scope
  Scope1 : Scope
  Sum5 : Sum  Inputs=|+-
  Switch : Switch  Criteria=u2 > Threshold  ZeroCross=off  SaturateOnIntegerOverflow=off  InputSameDT=off
  To Workspace1 : ToWorkspace  VariableName=RLslipError  SaveFormat=Timeseries  SampleTime=-1
  fl Slip : ToWorkspace  VariableName=RLsr1  SampleTime=-1
  Allowable Torque : Outport
  wires:
  Constant/1 -> Switch/3
  slipTarget/1 -> MATLAB Function/2(SlipTarget)
  MATLAB Function/1(enable) -> Switch/2, Scope/1
  slip Ratio/1 -> fl Slip/1, MATLAB Function/1(actualSlip), Sum5/2
  Switch/1 -> Allowable Torque/1
  MATLAB Function/2(setpoint) -> Sum5/1
  Sum5/1 -> To Workspace1/1, PID Controller5/1  "slip error"
  PID Controller5/1 -> Scope1/1, Switch/1

== system TorqueVectoring_6_1/Traction Control/RR ==
  slip Ratio : Inport
  slipTarget : Inport  Port=2
  Constant : Constant  Value=0
  MATLAB Function : MATLAB Function  TreatAsAtomicUnit=on
  PID Controller5 : slpidlib/PID Controller  Controller=PID  Form=Parallel  TimeDomain=Continuous-time  UseExternalTs=off  SampleTime=-1  IntegratorMethod=Forward Euler  FilterMethod=Forward Euler  ControllerParametersSource=internal  P=Kp_slip  I=Ki_slip  UseKiTs=off  D=Kd_slip  N=100  UseFilter=on  TunerSelectOption=Transfer Function Based (PID Tuner App)  ZeroCross=off  InitialConditionSource=internal  InitialConditionForIntegrator=0  InitialConditionForFilter=0  DifferentiatorICPrevScaledInput=0  ExternalReset=none  TrackingMode=off  Kt=1  LimitOutput=off  SatLimitsSource=internal  UpperSaturationLimit=slip_windupUpper  LowerSaturationLimit=slip_windupLower  LinearizeAsGain=on  AntiWindupMode=clamping  Kb=1  LimitIntegrator=off  UpperIntegratorSaturationLimit=inf  LowerIntegratorSaturationLimit=-inf  POutMin=[]  POutMax=[]  IOutMin=[]  IOutMax=[]  DOutMin=[]  DOutMax=[]  NOutMin=[]  NOutMax=[]  SumOutMin=[]  SumOutMax=[]  SaturationOutMin=[]  SaturationOutMax=[]  PParamMin=[]  PParamMax=[]  IParamMin=[]  IParamMax=[]  DParamMin=[]  DParamMax=[]  NParamMin=[]  NParamMax=[]  KbParamMin=[]  KbParamMax=[]  KtParamMin=[]  KtParamMax=[]  KbOutMin=[]  KbOutMax=[]  KtOutMin=[]  KtOutMax=[]  IntegratorOutMin=[]  IntegratorOutMax=[]  FilterOutMin=[]  FilterOutMax=[]  SumI1OutMin=[]  SumI1OutMax=[]  SumI2OutMin=[]  SumI2OutMax=[]  SumI3OutMin=[]  SumI3OutMax=[]  SumI4OutMin=[]  SumI4OutMax=[]  SumDOutMin=[]  SumDOutMax=[]  DifferentiatorOutMin=[]  DifferentiatorOutMax=[]  FilterDiffOutCoefMin=[]  FilterDiffOutCoefMax=[]  ReciprocalOutMin=[]  ReciprocalOutMax=[]  SumDenOutMin=[]  SumDenOutMax=[]  SumNumOutMin=[]  SumNumOutMax=[]  DivideOutMin=[]  DivideOutMax=[]  UdiffTsProdOutMin=[]  UdiffTsProdOutMax=[]  NTsProdOutMin=[]  NTsProdOutMax=[]  UintegralTsProdOutMin=[]  UintegralTsProdOutMax=[]  UngainTsProdOutMin=[]  UngainTsProdOutMax=[]  ClampingZeroOutDataTypeStr=Inherit: Inherit via back propagation  ClampingZeroOutMin=[]  ClampingZeroOutMax=[]  FilterDenConstantOutDataTypeStr=Inherit: Inherit via back propagation  FilterDenConstantOutMin=[]  FilterDenConstantOutMax=[]  PCopyOutDataTypeStr=Inherit: Inherit via back propagation  PCopyOutMin=[]  PCopyOutMax=[]  NCopyOutDataTypeStr=Inherit: Inherit via back propagation  NCopyOutMin=[]  NCopyOutMax=[]  IntegratorContinuousStateAttributes=''  IntegratorStateMustResolveToSignalObject=off  IntegratorRTWStateStorageClass=Auto  FilterContinuousStateAttributes=''  FilterStateMustResolveToSignalObject=off  FilterRTWStateStorageClass=Auto  ParallelPVariant=InternalParameters  IdealPVariant=Disabled  IVariant=InternalParameters  DVariant=InternalParameters  IntegratorVariant=Continuous  SatVariant=Disabled  AWVariant=Passthrough  PCopyVariant=Disabled  TRVariant=Disabled  FdbkBlocksVariant=Forward  IdealPFdbkVariant=Disabled  SatFdbkVariant=Disabled  DerivativeFilterVariant=ContFilter  NVariant=InternalParameters  NCopyVariant=Disabled  FilterICVariant=InternalICsFilter  IntegratorICVariant=InternalICs  ExternalResetVariant=Disabled  TRSumVariant=Passthrough  SumFdbkVariant=Disabled  SumVariant=Sum_PID  TsampFilterVariant=InternalTs  TsampNgainVariant=Passthrough  TsampIntegralVariant=Disabled_SignalSpec  ExternalSaturationOutDataTypeStr=Inherit: Same as second input
  Scope : Scope
  Scope1 : Scope
  Sum5 : Sum  Inputs=|+-
  Switch : Switch  Criteria=u2 > Threshold  ZeroCross=off  SaturateOnIntegerOverflow=off  InputSameDT=off
  To Workspace1 : ToWorkspace  VariableName=RRslipError  SaveFormat=Timeseries  SampleTime=-1
  fl Slip : ToWorkspace  VariableName=RRsr1  SampleTime=-1
  Allowable Torque : Outport
  wires:
  Constant/1 -> Switch/3
  slipTarget/1 -> MATLAB Function/2(SlipTarget)
  MATLAB Function/1(enable) -> Switch/2, Scope/1
  slip Ratio/1 -> fl Slip/1, MATLAB Function/1(actualSlip), Sum5/2
  Switch/1 -> Allowable Torque/1
  MATLAB Function/2(setpoint) -> Sum5/1
  Sum5/1 -> To Workspace1/1, PID Controller5/1  "slip error"
  PID Controller5/1 -> Scope1/1, Switch/1

== system TorqueVectoring_6_1/Vehicle Dynamics Model/14 DOF MODEL ==
  note: Fxrl
  steer : Inport
  Vx (Initial) : Inport  Port=2
  TaFL : Inport  Port=3
  TaFR : Inport  Port=4
  TaRL : Inport  Port=5
  TaRR : Inport  Port=6
  Fz : Mux
  Steering ratio : Gain  Gain=1/21
  Subsys Handling : Subsystem
  Subsys Tire : Subsystem
  Subsys ride : Subsystem
  To Workspace1 : ToWorkspace  VariableName=xPosition  SampleTime=-1
  To Workspace2 : ToWorkspace  VariableName=yPosition  SampleTime=-1
  degree conversion : Subsystem
  ay : Outport
  yaw rate : Outport  Port=2
  roll angle : Outport  Port=3
  fl slip angle : Outport  Port=4
  fr slip angle : Outport  Port=5
  rl slip angle : Outport  Port=6
  rr slip angle : Outport  Port=7
  X : Outport  Port=8
  Y : Outport  Port=9
  fl Slip Ratio : Outport  Port=10
  fr Slip Ratio : Outport  Port=11
  rl Slip Ratio : Outport  Port=12
  rr Slip Ratio : Outport  Port=13
  Veh Velocity : Outport  Port=14
  Corner Fz : Outport  Port=15
  wires:
  degree conversion/1(alpha(rad)) -> Subsys Handling/1(delta)  "radians"
  Subsys ride/3(Fzfr) -> Subsys Tire/2(Fzfr), Fz/2
  Subsys ride/4(Fzrl) -> Subsys Tire/3(Fzrl), Fz/3
  Subsys ride/5(Fzrr) -> Fz/4, Subsys Tire/4(Fzrr)
  Subsys Handling/4(ax) -> Subsys ride/1(ax)
  Subsys Handling/6(Safl) -> fl Slip Ratio/1, Subsys Tire/5(Sfl)
  Subsys Handling/7(alpha fl) -> fl slip angle/1, Subsys Tire/6(alphafl)
  Subsys Handling/8(Safr) -> fr Slip Ratio/1, Subsys Tire/7(Sfr)
  Subsys Handling/9(alpha fr) -> fr slip angle/1, Subsys Tire/8(alphafr)
  Subsys Handling/10(Sarl) -> rl Slip Ratio/1, Subsys Tire/9(Srl)
  Subsys Handling/11(alpha rl) -> rl slip angle/1, Subsys Tire/10(alpharl)
  Subsys Handling/12(Sarr) -> rr Slip Ratio/1, Subsys Tire/11(Srr)
  Subsys Handling/13(alpha rr) -> Subsys Tire/12(alpharr), rr slip angle/1
  Subsys Tire/12(Mzrr) -> Subsys Handling/13(Mzrr)
  Subsys Tire/11(Mzrl) -> Subsys Handling/12(Mzrl)
  Subsys Tire/10(Mzfr) -> Subsys Handling/11(Mzfr)
  Subsys Tire/9(Mzfl) -> Subsys Handling/10(Mzfl)
  Subsys Tire/8(Fyrr) -> Subsys Handling/9(Fyrr)
  Subsys Tire/7(Fxrr) -> Subsys Handling/8(Fxrr)
  Subsys Tire/6(Fyrl) -> Subsys Handling/7(Fyrl)
  Subsys Tire/5(Fxrl) -> Subsys Handling/6(Fxrl)
  Subsys Tire/4(Fyfr) -> Subsys Handling/5(Fyfr)
  Subsys Tire/3(Fxfr) -> Subsys Handling/4(Fxfr)
  Subsys Tire/2(Fyfl) -> Subsys Handling/3(Fyfl)  "LatF fl"
  Subsys Tire/1(Fxfl) -> Subsys Handling/2(Fxfl)
  steer/1 -> Steering ratio/1
  Steering ratio/1 -> degree conversion/1(alpha(degree))  "deg"
  TaFL/1 -> Subsys Handling/15(TaFL)
  Subsys ride/1(phi) -> roll angle/1
  Subsys Handling/5(ay) -> ay/1, Subsys ride/2(ay)
  Subsys Handling/3(psi dot) -> yaw rate/1
  Subsys Handling/1(X) -> X/1, To Workspace1/1
  Subsys Handling/2(Y) -> To Workspace2/1, Y/1
  TaRL/1 -> Subsys Handling/16(TaRL)
  TaFR/1 -> Subsys Handling/17(TaFR)
  TaRR/1 -> Subsys Handling/18(TaRR)
  Subsys ride/2(Fzfl) -> Subsys Tire/1(Fzfl), Fz/1
  Vx (Initial)/1 -> Subsys Handling/14(Vx)
  Subsys Handling/14(Veh Velocity) -> Veh Velocity/1
  Fz/1 -> Corner Fz/1

== system TorqueVectoring_6_1/Vehicle Dynamics Model/Signal Builder ==
  Demux : Demux  Tag=STV Demux  Outputs=1
      settings: DisplayOption=none
  FromWs : FromWorkspace  Tag=STV FromWs  VariableName=tuvar
      SigBuilderData=|
      | common.afterFinalStr = 'Extrapolate'
      | common.sampleTime = 0
      | dataSet.timeRange = [0 10]
      | dataSet.name = 'Group 1'
      | sbobj.Groups.Name = 'Group 1'
      | sbobj.Groups.Signals.Name = 'Signal 1'
      | sbobj.Groups.Signals.XData = [0 10]
      | sbobj.Groups.Signals.YData = [-250 -250]
  Signal 1 : Outport  Tag=STV Outport
  wires:
  Demux/1 -> Signal 1/1
  FromWs/1 -> Demux/1

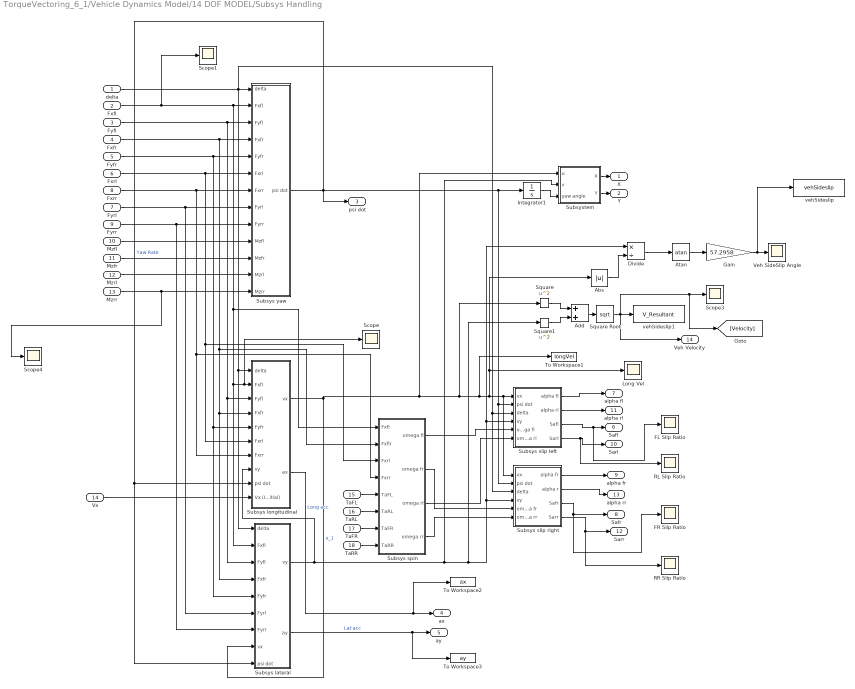
== system TorqueVectoring_6_1/Vehicle Dynamics Model/14 DOF MODEL/Subsys Handling ==
  delta : Inport
  Fxfl : Inport  Port=2
  Fyfl : Inport  Port=3
  Fxfr : Inport  Port=4
  Fyfr : Inport  Port=5
  Fxrl : Inport  Port=6
  Fyrl : Inport  Port=7
  Fxrr : Inport  Port=8
  Fyrr : Inport  Port=9
  Mzfl : Inport  Port=10
  Mzfr : Inport  Port=11
  Mzrl : Inport  Port=12
  Mzrr : Inport  Port=13
  Vx : Inport  Port=14
  TaFL : Inport  Port=15
  TaRL : Inport  Port=16
  TaFR : Inport  Port=17
  TaRR : Inport  Port=18
  Abs : Abs  SaturateOnIntegerOverflow=off
  Add : Sum
  Atan : Trigonometry  Operator=atan
  Divide : Product  Inputs=*/
  FL Slip Ratio : Scope
  FR Slip Ratio : Scope
  Gain : Gain  Gain=57.2958
  Integrator1 : Integrator
  Long Vel : Scope
  RL Slip Ratio : Scope
  RR Slip Ratio : Scope
  Scope{,1,3..4} (4 alike) : Scope
  Square : Math  Operator=square
  Square Root : Sqrt
  Square1 : Math  Operator=square
  Subsys lateral : Subsystem
  Subsys longitudinal : Subsystem
  "Subsys slip left " : Subsystem
  Subsys slip right : Subsystem
  Subsys spin : Subsystem
  "Subsys yaw " : Subsystem
  Subsystem : Subsystem
  To Workspace1 : ToWorkspace  VariableName=longVel  SampleTime=-1
  To Workspace2 : ToWorkspace  VariableName=ax  SaveFormat=Timeseries  SampleTime=-1
  To Workspace3 : ToWorkspace  VariableName=ay  SaveFormat=Timeseries  SampleTime=-1
  Veh SideSlip Angle : Scope
  vehSideslip : ToWorkspace  VariableName=vehSideslip  SampleTime=-1
  vehSideslip1 : ToWorkspace  VariableName=V_Resultant  SaveFormat=Timeseries  SampleTime=-1
  X : Outport
  Y : Outport  Port=2
  psi dot : Outport  Port=3
  ax : Outport  Port=4
  ay : Outport  Port=5
  Safl : Outport  Port=6
  alpha fl : Outport  Port=7
  Safr : Outport  Port=8
  alpha fr : Outport  Port=9
  Sarl : Outport  Port=10
  alpha rl : Outport  Port=11
  Sarr : Outport  Port=12
  alpha rr : Outport  Port=13
  Veh Velocity : Outport  Port=14
  wires:
  Subsys lateral/2(ay) -> To Workspace3/1, ay/1  "Lat acc"
  Subsys longitudinal/2(ax) -> To Workspace2/1, ax/1  "Long acc"
  TaFL/1 -> Subsys spin/5(TaFL)
  Fxrr/1 -> Subsys longitudinal/7(Fxrr), Subsys spin/4(Fxrr), "Subsys yaw "/7(Fxrr)
  "Subsys slip left "/1(alpha fl) -> alpha fl/1
  Subsys slip right/1(alpha fr) -> alpha fr/1
  Subsys slip right/2(alpha r) -> alpha rr/1
  Subsys spin/1(omega fl) -> "Subsys slip left "/5(omega fl)
  Subsys spin/4(omega rr) -> Subsys slip right/6(omega rr)
  Subsys longitudinal/1(vx) -> Square/1, To Workspace1/1, Abs/1, Long Vel/1, "Subsys slip left "/1(vx), Subsys slip right/1(vx), Subsystem/1(u), Subsys lateral/8(vx)  "x_1"
  "Subsys slip left "/2(alpha rl) -> alpha rl/1
  delta/1 -> "Subsys yaw "/1(delta), Subsys longitudinal/1(delta), Subsys lateral/1(delta), "Subsys slip left "/3(delta), Subsys slip right/3(delta)
  Fxfl/1 -> Scope1/1, Scope/1, Subsys longitudinal/2(Fxfl), Subsys lateral/2(Fxfl), Subsys spin/1(Fxfl), "Subsys yaw "/2(Fxfl)
  Fyfl/1 -> "Subsys yaw "/3(Fyfl), Subsys longitudinal/3(Fyfl), Subsys lateral/3(Fyfl)
  Fxfr/1 -> Subsys lateral/4(Fxfr), Subsys longitudinal/4(Fxfr), Subsys spin/2(Fxflr), "Subsys yaw "/4(Fxfr)
  Fyfr/1 -> "Subsys yaw "/5(Fyfr), Subsys lateral/5(Fyfr), Subsys longitudinal/5(Fyfr)
  Fxrl/1 -> Subsys longitudinal/6(Fxrl), Subsys spin/3(Fxrl), "Subsys yaw "/6(Fxrl)
  Fyrl/1 -> "Subsys yaw "/8(Fyrl), Subsys lateral/6(Fyrl)
  Fyrr/1 -> "Subsys yaw "/9(Fyrr), Subsys lateral/7(Fyrr)
  "Subsys yaw "/1(psi dot) -> psi dot/1, Subsys lateral/9("psi dot "), Subsys longitudinal/9("psi dot "), "Subsys slip left "/2(psi dot), Subsys slip right/2(psi dot), Integrator1/1  "Yaw Rate"
  Subsys lateral/1(vy) -> Subsys longitudinal/8(vy), Divide/1, "Subsys slip left "/4(vy), Subsys slip right/4(vy), Square1/1, Subsystem/2(v)
  Mzfl/1 -> "Subsys yaw "/10(Mzfl)
  Mzrr/1 -> Scope4/1, "Subsys yaw "/13(Mzrr)
  Mzrl/1 -> "Subsys yaw "/12(Mzrl)
  Mzfr/1 -> "Subsys yaw "/11(Mzfr)
  Subsys spin/2(omega fr) -> Subsys slip right/5(omega fr)
  Subsys spin/3(omega rl) -> "Subsys slip left "/6(omega rl)
  Vx/1 -> Subsys longitudinal/10(Vx (Initial))
  Integrator1/1 -> Subsystem/3(yaw angle)
  Subsystem/1(X) -> X/1
  Subsystem/2(Y) -> Y/1
  "Subsys slip left "/4(Sarl) -> RL Slip Ratio/1, Sarl/1
  Subsys slip right/4(Sarr) -> RR Slip Ratio/1, Sarr/1
  TaRL/1 -> Subsys spin/6(TaRL)
  TaFR/1 -> Subsys spin/7(TaFR)
  TaRR/1 -> Subsys spin/8(TaRR)
  "Subsys slip left "/3(Safl) -> FL Slip Ratio/1, Safl/1
  Divide/1 -> Atan/1
  Atan/1 -> Gain/1
  Abs/1 -> Divide/2
  Gain/1 -> vehSideslip/1, Veh SideSlip Angle/1
  Add/1 -> Square Root/1
  Square/1 -> Add/1
  Square1/1 -> Add/2
  Square Root/1 -> [Velocity], Scope3/1, Veh Velocity/1, vehSideslip1/1
  Subsys slip right/3(Safr) -> Safr/1, FR Slip Ratio/1
